simulink model "FOC"  (R2023b)
settings: Solver=VariableStepAuto  StartTime=0.0  StopTime=10  RelTol=1e-3
libraries: spsAsynchronousMachineSIUnitsLib x1, spsDCVoltageSourceLib x1, spsThreePhaseVIMeasurementLib x1, spsUniversalBridgeLib x1, sps_lib x1
settings Model: Creator=LEGION  LastModifiedBy=86189
settings SolverCC: AlgebraicLoopSolver=TrustRegion
settings DebuggingCC: ArithmeticOperatorsInVariantConditions=warning
settings SFSimCC: CustomCodeUndefinedFunction=UseInterfaceOnly

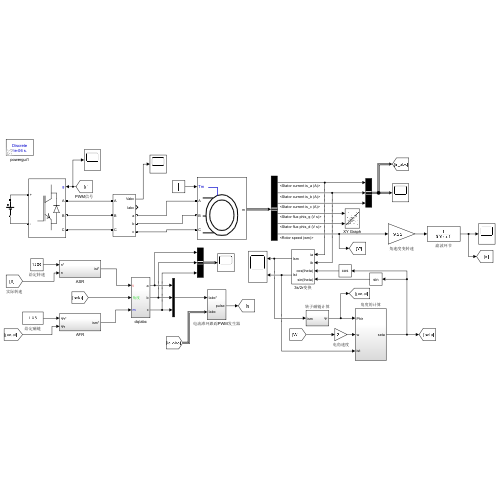
[thumbnail: Simulink's stored preview of the top-level diagram]
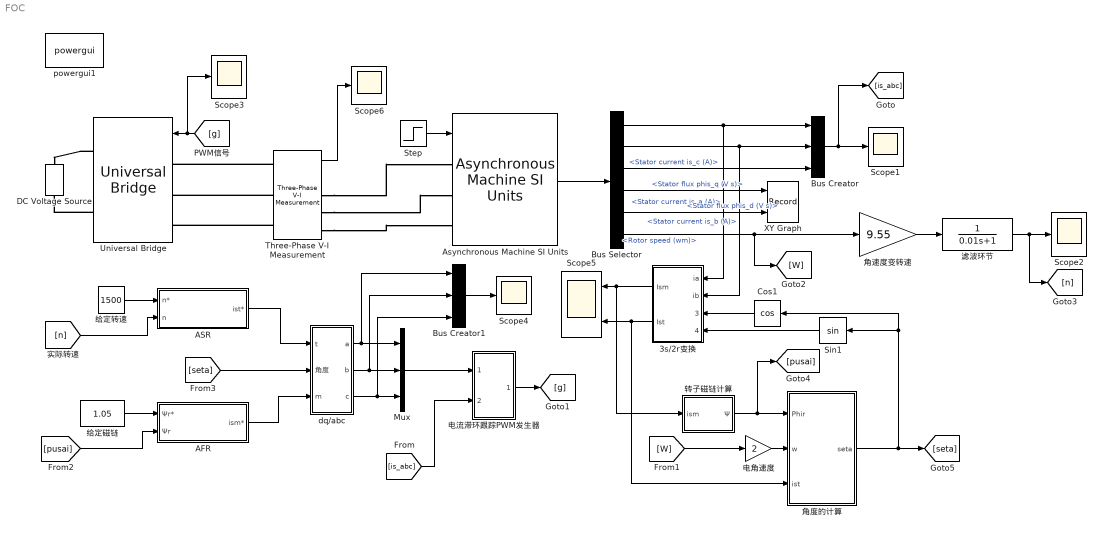
== system FOC ==
  3s/2r变换 : Subsystem
  AFR : Subsystem
  ASR : Subsystem
  Asynchronous Machine SI Units : spsAsynchronousMachineSIUnitsLib/Asynchronous Machine SI Units  RotorType=Squirrel-cage  PresetModel=No  MechanicalLoad=Torque Tm  ShowDetailedParameters=on  ReferenceFrame=Rotor  Units=SI  MeasurementBus=off  NominalParameters=[1.1e+05 400 50]  VoltageRatio=1  Stator=[0.02155 0.000226]  Rotor=[0.01231 0.000226]  Cage1=[0.4155 0.002066]  Cage2=[0.4168 0.0003495]  Lm=0.01038  Mechanical=[2.3 0.05421 2]  PolePairs=2  InitialConditions=[1 0 0 0 0 0 0 0]  SimulateSaturation=off  Saturation=[14.03593122, 27.81365428, 53.79336849, 72.68890987, 97.98006896, 148.6815601, 215.7428561, 302.9841135, 428.7778367 ; 230, 322, 414, 460, 506, 552, 598, 644, 690]  LoadFlowParameters=1492000  TsPowergui=0  TsBlock=-1  IterativeModel=Trapezoidal non iterative  IterativeDiscreteModel=Trapezoidal non iterative  Pmec=1.492e+006
  Bus Creator : BusCreator  Inputs=3
  Bus Creator1 : BusCreator  Inputs=3
  Bus Selector : BusSelector  OutputSignals=Stator measurements.Stator current is_a (A),Stator measurements.Stator current is_b (A),Stator measurements.Stator current is_c (A),Stator measurements.Stator flux phis_q (V s),Stator measurements.Stator flux phis_d (V s),Mechanical.Rotor speed (wm)
  Cos1 : Trigonometry  Operator=cos
  DC Voltage Source : spsDCVoltageSourceLib/DC Voltage Source  Amplitude=513  Measurements=None
  Mux : Mux  Inputs=3
  Scope{1..4,6} (5 alike) : Scope
  Scope5 : Scope  NumInputPorts=2
  Sin1 : Trigonometry
  Step : Step  Time=9  Before=706  After=300  SampleTime=0
  Three-Phase V-I Measurement : spsThreePhaseVIMeasurementLib/Three-Phase V-I Measurement  VoltageMeasurement=phase-to-phase  SetLabelV=off  LabelV=Vabc  Vpu=off  VpuLL=off  CurrentMeasurement=yes  SetLabelI=off  LabelI=Iabc  Ipu=off  Pbase=100e6  Vbase=500e3  OutputType=Complex  PhasorSimulation=off  PSBequivalent=0
  Universal Bridge : spsUniversalBridgeLib/Universal Bridge  Arms=3  SnubberResistance=1e5  SnubberCapacitance=inf  Device=IGBT / Diodes  Ron=1e-3  Lon=0  ForwardVoltages="[  0  0  ]"  ForwardVoltage=0  GTOparameters=[ 10e-6 , 20e-6 ]  IGBTparameters=[ 1e-6 , 2e-6 ]  Measurements=None  Measurements_2=None  converterType=Rectifier
  XY Graph : Record  FileSettingsInternal="{\"entries\":[{\"content\":{\"excelSettings\":{\"content\":{},\"type\":\"Streamout.ExcelSettings\"}},\"type\":\"Streamout.FileSettingStorage\",\"uuid\":\"\"}],\"packageUris\":[\"http:\\/\\/schema.mathworks.com\\/mf0\\/streamout_blocks\\/R2020a\"],\"version\":\"1.0\"}"  Layout=[1 1]  SignalsInternal="{\"entries\":[{\"content\":{\"signals\":[{\"content\":{\"blockPath\":[],\"dimensions\":[1],\"domain\":\"\",\"lineColor\":\"#a2142f\",\"plots\":[1],\"port\":1,\"sid\":[\"\"],\"signalID\":6612,\"signalName\":\"<Stator flux phis_q (V s)>\"},\"type\":\"RecordBlkView.Signal\",\"uuid\":\"\"},{\"content\":{\"blockPath\":[],\"dimensions\":[1],\"domain\":\"\",\"lineColor\":\"#139fff\",\"plots\":[1],\"port\":2,\"sid\":[\"\"],\"signalID\":6616,\"signalName\":\"<Stator flux phis_d (V s)>\"},\"type\":\"RecordBlkView.Signal\",\"uuid\":\"\"}]},\"type\":\"RecordBlkView.InputSignals\",\"uuid\":\"\"}],\"packageUris\":[\"http:\\/\\/schema.mathworks.com\\/mf0\\/streamout_blocks\\/R2020a\"],\"version\":\"1.0\"}"  VisualizationBindings="{\"xyplotplugin\":{\"info\":[{\"series\":[{\"bindingParametersList\":[{\"parameter\":\"X-Axis\",\"signalID\":6612,\"signalName\":\"<Stator flux phis_q (V s)>\"},{\"parameter\":\"Y-Axis\",\"signalID\":6616,\"signalName\":\"<Stator flux phis_d (V s)>\"}],\"seriesID\":52085}],\"subplotID\":1}]}}"  CompatibilityTag=XY  st=-1
  dq/abc : Subsystem
  powergui1 : sps_lib/powergui  Priority=1  SimulationMode=Discrete  SampleTime=50e-7  frequency=60  Iterations=50  frequencyindice=50  Pbase=100e6  ErrMax=1e-4  UnitsV=kV  UnitsW=MW  buscounter=0  FunctionMessages=off  echomessages=off  EnableUseOfTLC=off  CurrentSourceSwitches=off  DisableSnubberDevices=off  DisableRonSwitches=off  DisableVfSwitches=off  DisplayEquations=off  AutomaticDiscreteSolvers=off  SolverType=Tustin/Backward Euler (TBE)  Interpol=off  ExternalGateDelay=off  methode=off  Ts=10  x0status=blocks  SPID=off  SwTol=0  HookPort=off  NonlinearTolerance=1e-4  nMaxIteration=100  ContinueOnMaxIteration=off  RestoreLinks=warning  ResistiveCurrentMeasurement=off  Frange=[0:2:500]  Ylog=off  Xlog=on  ShowGrid=off  save=off  variable=ZData  structure=0  ZoomFFT=off  StartTime=0.0  cycles=1  DisplayStyle=1  fundamental=60  FreqAxis=off  MaxFrequency=1000  frequencyindicesteady=1  RmsSteady=1  display=off
  滤波环节 : TransferFcn  Denominator=[0.01 1]
  电流滞环跟踪PWM发生器 : Subsystem
  电角速度 : Gain  Gain=2
  给定磁链 : Constant  Value=1.05
  给定转速 : Constant  Value=1500
  角度的计算 : Subsystem
  角速度变转速 : Gain  Gain=9.55
  转子磁链计算 : Subsystem
  wires:
  dq/abc/1(a) -> Bus Creator1/1, Mux/1
  dq/abc/3(c) -> Bus Creator1/3, Mux/3
  给定磁链/1 -> AFR/1(Ψr*)
  Bus Selector/3 -> Bus Creator/3  "<Stator current is_c (A)>"
  dq/abc/2(b) -> Bus Creator1/2, Mux/2
  ASR/1(ist*) -> dq/abc/1(t)
  Bus Selector/2 -> 3s/2r变换/2(ib), Bus Creator/2  "<Stator current is_b (A)>"
  Step/1 -> Asynchronous Machine SI Units/1
  Bus Selector/1 -> 3s/2r变换/1(ia), Bus Creator/1  "<Stator current is_a (A)>"
  给定转速/1 -> ASR/1(n*)
  Bus Creator/1 -> Scope1/1, [is_abc]
  Bus Selector/6 -> [W], 角速度变转速/1  "<Rotor speed (wm)>"
  Asynchronous Machine SI Units/1 -> Bus Selector/1
  AFR/1(ism*) -> dq/abc/3(m)
  [g] -> Scope3/1, Universal Bridge/1
  Bus Selector/4 -> XY Graph/1  "<Stator flux phis_q (V s)>"
  角速度变转速/1 -> 滤波环节/1
  滤波环节/1 -> Scope2/1, [n]
  [n] -> ASR/2(n)
  3s/2r变换/2(Ist) -> 角度的计算/3(ist), Scope5/2
  3s/2r变换/1(Ism) -> 转子磁链计算/1(ism), Scope5/1
  电角速度/1 -> 角度的计算/2(w)
  [W] -> 电角速度/1
  转子磁链计算/1(Ψ) -> [pusai], 角度的计算/1(Phir)
  Cos1/1 -> 3s/2r变换/3(cos(theta))
  Sin1/1 -> 3s/2r变换/4(sin(theta))
  角度的计算/1(seta) -> [seta], Sin1/1, Cos1/1
  [seta] -> dq/abc/2(角度)
  [pusai] -> AFR/2(Ψr)
  Three-Phase V-I Measurement/1 -> Scope6/1
  Mux/1 -> 电流滞环跟踪PWM发生器/1(Iabc*)
  电流滞环跟踪PWM发生器/1(pulse) -> [g]
  [is_abc] -> 电流滞环跟踪PWM发生器/2(Iabc)
  Bus Selector/5 -> XY Graph/2  "<Stator flux phis_d (V s)>"
  Bus Creator1/1 -> Scope4/1
  connections:
  Universal Bridge/RConn2 -- DC Voltage Source/LConn1
  Universal Bridge/RConn1 -- DC Voltage Source/RConn1
  Three-Phase V-I Measurement/LConn1 -- Universal Bridge/LConn1
  Three-Phase V-I Measurement/LConn2 -- Universal Bridge/LConn2
  Three-Phase V-I Measurement/LConn3 -- Universal Bridge/LConn3
  Three-Phase V-I Measurement/RConn1 -- Asynchronous Machine SI Units/LConn1
  Three-Phase V-I Measurement/RConn2 -- Asynchronous Machine SI Units/LConn2
  Three-Phase V-I Measurement/RConn3 -- Asynchronous Machine SI Units/LConn3

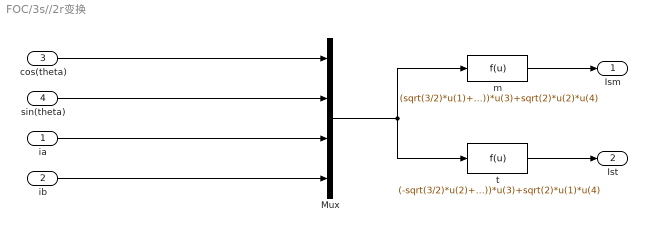
== system FOC/3s//2r变换 ==
  ia : Inport
  ib : Inport  Port=2
  cos(theta) : Inport  Port=3
  sin(theta) : Inport  Port=4
  Mux : Mux
  m : Fcn  Expr=(sqrt(3/2)*u(1)+sqrt(1/2)*u(2))*u(3)+sqrt(2)*u(2)*u(4)
  t : Fcn  Expr=(-sqrt(3/2)*u(2)+sqrt(1/2)*u(1))*u(3)+sqrt(2)*u(1)*u(4)
  Ism : Outport
  Ist : Outport  Port=2
  wires:
  ib/1 -> Mux/4
  t/1 -> Ist/1
  ia/1 -> Mux/3
  sin(theta)/1 -> Mux/2
  Mux/1 -> t/1, m/1
  m/1 -> Ism/1
  cos(theta)/1 -> Mux/1

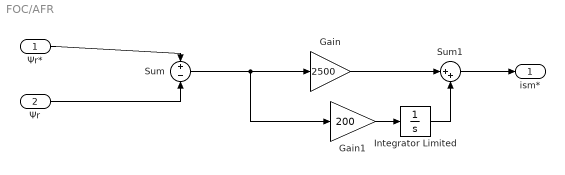
== system FOC/AFR ==
  Ψr* : Inport
  Ψr : Inport  Port=2
  Gain : Gain  Gain=2500
  Gain1 : Gain  Gain=200
  Integrator Limited : Integrator  LimitOutput=on  UpperSaturationLimit=100  LowerSaturationLimit=-100
  Sum : Sum  Inputs=+-
  Sum1 : Sum  Inputs=|++
  ism* : Outport
  wires:
  Integrator Limited/1 -> Sum1/2
  Gain/1 -> Sum1/1
  Gain1/1 -> Integrator Limited/1
  Sum/1 -> Gain/1, Gain1/1
  Ψr/1 -> Sum/2
  Ψr*/1 -> Sum/1
  Sum1/1 -> ism*/1

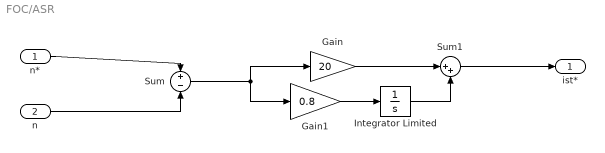
== system FOC/ASR ==
  n* : Inport
  n : Inport  Port=2
  Gain : Gain  Gain=20
  Gain1 : Gain  Gain=0.8
  Integrator Limited : Integrator  LimitOutput=on  UpperSaturationLimit=80  LowerSaturationLimit=-80
  Sum : Sum  Inputs=+-
  Sum1 : Sum  Inputs=|++
  ist* : Outport
  wires:
  Integrator Limited/1 -> Sum1/2
  Gain/1 -> Sum1/1
  Gain1/1 -> Integrator Limited/1
  Sum/1 -> Gain/1, Gain1/1
  n/1 -> Sum/2
  n*/1 -> Sum/1
  Sum1/1 -> ist*/1

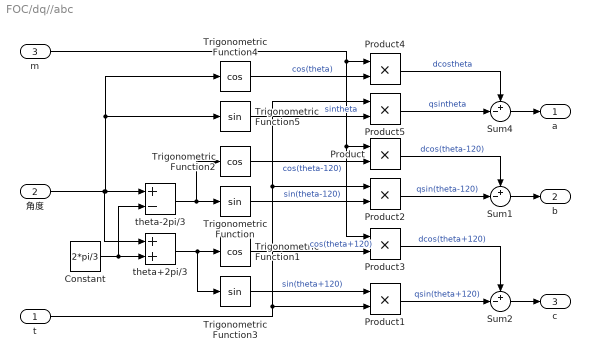
== system FOC/dq//abc ==
  t : Inport
  角度 : Inport  Port=2
  m : Inport  Port=3
  Constant : Constant  Value=2*pi/3
  Product{,1..5} (6 alike) : Product
  Sum1 : Sum  Inputs=+-|
  Sum2 : Sum  Inputs=+-|
  Sum4 : Sum  Inputs=+-|
  Trigonometric Function : Trigonometry
  Trigonometric Function1 : Trigonometry  Operator=cos
  Trigonometric Function2 : Trigonometry  Operator=cos
  Trigonometric Function3 : Trigonometry
  Trigonometric Function4 : Trigonometry  Operator=cos
  Trigonometric Function5 : Trigonometry
  theta+2pi/3 : Sum
  theta-2pi/3 : Sum  Inputs=+-
  a : Outport  VectorParamsAs1DForOutWhenUnconnected=off
  b : Outport  Port=2  VectorParamsAs1DForOutWhenUnconnected=off
  c : Outport  Port=3  VectorParamsAs1DForOutWhenUnconnected=off
  wires:
  Trigonometric Function5/1 -> Product5/2  "sintheta"
  Product/1 -> Sum1/1  "dcos(theta-120)"
  Trigonometric Function1/1 -> Product3/2  "cos(theta+120)"
  Product3/1 -> Sum2/1  "dcos(theta+120)"
  m/1 -> Product/1, Product3/1, Product4/1
  Constant/1 -> theta+2pi/3/2, theta-2pi/3/2
  角度/1 -> Trigonometric Function4/1, Trigonometric Function5/1, theta-2pi/3/1, theta+2pi/3/1
  theta+2pi/3/1 -> Trigonometric Function3/1, Trigonometric Function1/1
  t/1 -> Product5/1, Product2/1, Product1/2
  Trigonometric Function/1 -> Product2/2  "sin(theta-120)"
  Product4/1 -> Sum4/1  "dcostheta"
  Product5/1 -> Sum4/2  "qsintheta"
  theta-2pi/3/1 -> Trigonometric Function2/1, Trigonometric Function/1
  Product1/1 -> Sum2/2  "qsin(theta+120)"
  Trigonometric Function2/1 -> Product/2  "cos(theta-120)"
  Sum4/1 -> a/1
  Sum1/1 -> b/1
  Trigonometric Function4/1 -> Product4/2  "cos(theta)"
  Trigonometric Function3/1 -> Product1/1  "sin(theta+120)"
  Product2/1 -> Sum1/2  "qsin(theta-120)"
  Sum2/1 -> c/1

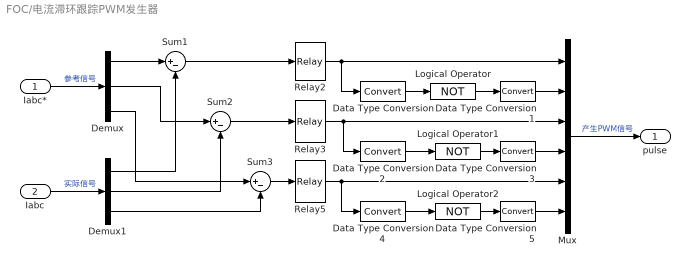
== system FOC/电流滞环跟踪PWM发生器 ==
  Iabc* : Inport
  Iabc : Inport  Port=2
  Data Type Conversion{,1..5} (6 alike) : DataTypeConversion  SaturateOnIntegerOverflow=off  RndMeth=Floor
  Demux : Demux  Outputs=3
  Demux1 : Demux  Outputs=3
  Logical Operator : Logic  Operator=NOT  Inputs=1  AllPortsSameDT=off
  Logical Operator1 : Logic  Operator=NOT  Inputs=1  AllPortsSameDT=off
  Logical Operator2 : Logic  Operator=NOT  Inputs=1  AllPortsSameDT=off
  Mux : Mux  Inputs=6
  Relay2 : Relay  OnSwitchValue=0.2  OffSwitchValue=-0.2  ZeroCross=off
  Relay3 : Relay  OnSwitchValue=0.2  OffSwitchValue=-0.2  ZeroCross=off
  Relay5 : Relay  OnSwitchValue=0.2  OffSwitchValue=-0.2  ZeroCross=off
  Sum1 : Sum  Inputs=|+-
  Sum2 : Sum  Inputs=|+-
  Sum3 : Sum  Inputs=|+-
  pulse : Outport  VectorParamsAs1DForOutWhenUnconnected=off
  wires:
  Relay2/1 -> Data Type Conversion/1, Mux/1
  Data Type Conversion/1 -> Logical Operator/1
  Logical Operator/1 -> Data Type Conversion1/1
  Data Type Conversion1/1 -> Mux/2
  Mux/1 -> pulse/1  "产生PWM信号"
  Sum1/1 -> Relay2/1
  Demux/1 -> Sum1/1
  Demux1/3 -> Sum3/2
  Iabc/1 -> Demux1/1  "实际信号"
  Iabc*/1 -> Demux/1  "参考信号"
  Sum2/1 -> Relay3/1
  Logical Operator1/1 -> Data Type Conversion3/1
  Data Type Conversion3/1 -> Mux/4
  Data Type Conversion2/1 -> Logical Operator1/1
  Relay3/1 -> Data Type Conversion2/1, Mux/3
  Logical Operator2/1 -> Data Type Conversion5/1
  Data Type Conversion5/1 -> Mux/6
  Data Type Conversion4/1 -> Logical Operator2/1
  Relay5/1 -> Data Type Conversion4/1, Mux/5
  Sum3/1 -> Relay5/1
  Demux/2 -> Sum2/1
  Demux1/1 -> Sum1/2
  Demux1/2 -> Sum2/2
  Demux/3 -> Sum3/1

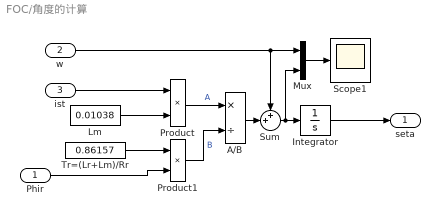
== system FOC/角度的计算 ==
  Phir : Inport
  w : Inport  Port=2
  ist : Inport  Port=3
  A/B : Product  Inputs=*/
  Integrator : Integrator
  Lm : Constant  Value=0.01038
  Mux : Mux  Inputs=2
  Product : Product
  Product1 : Product
  Scope1 : Scope
  Sum : Sum  Inputs=++|
  Tr=(Lr+Lm)/Rr : Constant  Value=0.86157
  seta : Outport  VectorParamsAs1DForOutWhenUnconnected=off
  wires:
  ist/1 -> Product/1
  w/1 -> Sum/1, Mux/1
  Product/1 -> A/B/1  "A"
  Sum/1 -> Mux/2, Integrator/1
  Integrator/1 -> seta/1
  Product1/1 -> A/B/2  "B"
  Lm/1 -> Product/2
  A/B/1 -> Sum/2
  Phir/1 -> Product1/2
  Tr=(Lr+Lm)/Rr/1 -> Product1/1
  Mux/1 -> Scope1/1

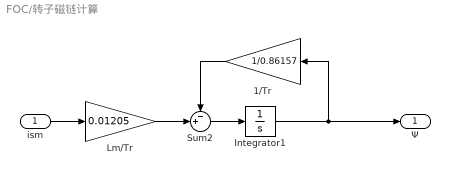
== system FOC/转子磁链计算 ==
  ism : Inport
  1/Tr : Gain  Gain=1/0.86157
  Integrator1 : Integrator  InitialCondition=1e-5
  Lm/Tr : Gain  Gain=0.01205
  Sum2 : Sum  Inputs=-+|
  Ψ : Outport  VectorParamsAs1DForOutWhenUnconnected=off
  wires:
  Sum2/1 -> Integrator1/1
  Integrator1/1 -> Ψ/1, 1/Tr/1
  ism/1 -> Lm/Tr/1
  Lm/Tr/1 -> Sum2/2
  1/Tr/1 -> Sum2/1
